simulink model "punto3_Fonseca"  (R2024a)
settings: Solver=VariableStepAuto  StartTime=0.0  StopTime=100  RelTol=1e-3
values from neighbouring files (symbols this model uses):
  G1 = 3    [punto_3_Coeficientes.m]
  G2 = 2*s + 1    [punto_3_Coeficientes.m]
  G3 = s^2 + A*s + 12    [punto_3_Coeficientes.m]
  G4 = -C    (= -4)    [punto_3_Coeficientes.m]
  G5 = -0.1    [punto_3_Coeficientes.m]
  G6 = s    [punto_3_Coeficientes.m]
  H1 = s^2 + C*s + 5    [punto_3_Coeficientes.m]
  H2 = B*s - 1    [punto_3_Coeficientes.m]
libraries: cstblocks x1
settings Model: Creator=Usuario  LastModifiedBy=Usuario

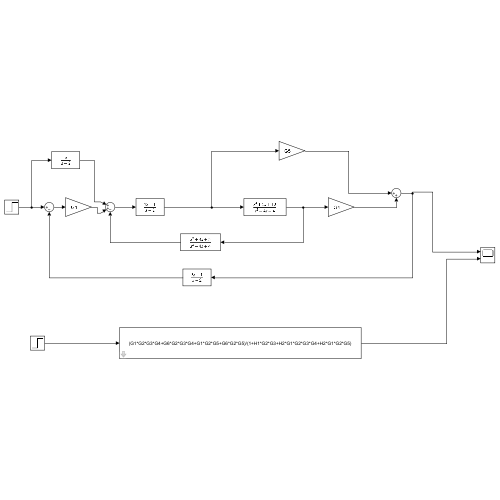
[thumbnail: Simulink's stored preview of the top-level diagram]
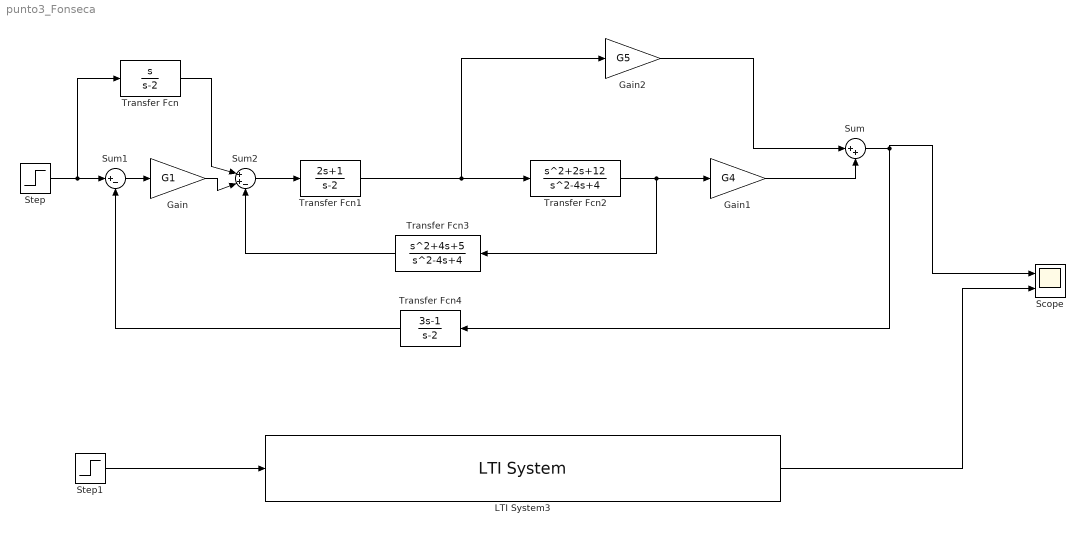
== system punto3_Fonseca ==
  Gain : Gain  Gain=G1
  Gain1 : Gain  Gain=G4
  Gain2 : Gain  Gain=G5
  LTI System3 : cstblocks/LTI System  sys=(G1*G2*G3*G4+G6*G2*G3*G4+G1*G2*G5+G6*G2*G5)/(1+H1*G2*G3+H2*G1*G2*G3*G4+H2*G1*G2*G5)  IC=[]  PadeOrder=0
  Scope : Scope  NumInputPorts=2
  Step : Step  SampleTime=0
  Step1 : Step  SampleTime=0
  Sum : Sum  Inputs=|++
  Sum1 : Sum  Inputs=|+-
  Sum2 : Sum  Inputs=|++-
  Transfer Fcn : TransferFcn  Numerator=[1 0]  Denominator=[1 -2]
  Transfer Fcn1 : TransferFcn  Numerator=[2 1]  Denominator=[1 -2]
  Transfer Fcn2 : TransferFcn  Numerator=[1 2 12]  Denominator=[1 -4 4]
  Transfer Fcn3 : TransferFcn  Numerator=[1 4 5]  Denominator=[1 -4 4]
  Transfer Fcn4 : TransferFcn  Numerator=[3 -1]  Denominator=[1 -2]
  wires:
  Step/1 -> Transfer Fcn/1, Sum1/1
  Sum1/1 -> Gain/1
  Transfer Fcn1/1 -> Transfer Fcn2/1, Gain2/1
  Gain/1 -> Sum2/2
  Transfer Fcn/1 -> Sum2/1
  Sum2/1 -> Transfer Fcn1/1
  Gain2/1 -> Sum/1
  Transfer Fcn2/1 -> Transfer Fcn3/1, Gain1/1
  Gain1/1 -> Sum/2
  Transfer Fcn3/1 -> Sum2/3
  Transfer Fcn4/1 -> Sum1/2
  Step1/1 -> LTI System3/1
  LTI System3/1 -> Scope/2
  Sum/1 -> Transfer Fcn4/1, Scope/1
